simulink model "SimulacionControl9"  (R2022b)
settings: Solver=VariableStepAuto  StartTime=0.0  StopTime=20  RelTol=1e-3
undefined symbols (not defined in the file): Cdifuso9
libraries: fuzblock x1
settings Model: Creator=PC-LUISMIGUEL  LastModifiedBy=David

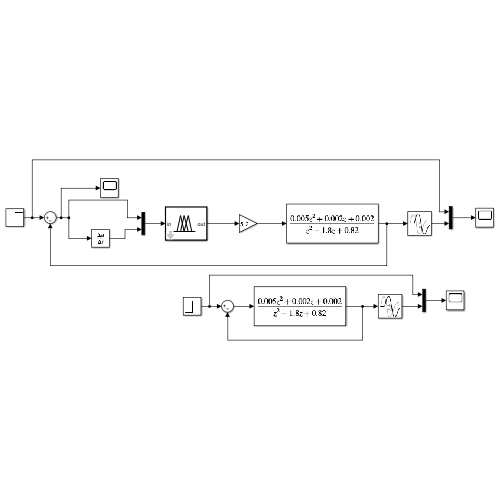
[thumbnail: Simulink's stored preview of the top-level diagram]
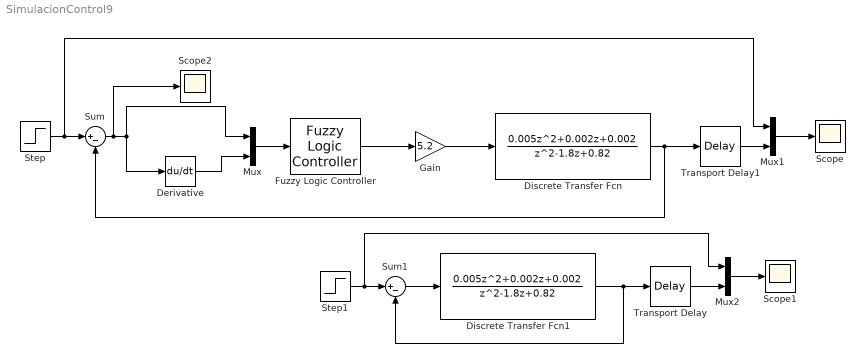
== system SimulacionControl9 ==
  Derivative : Derivative
  Discrete Transfer Fcn : DiscreteTransferFcn  Numerator=[0.005 0.002 0.002]  Denominator=[1 -1.8 0.82]  SampleTime=0.1
  Discrete Transfer Fcn1 : DiscreteTransferFcn  Numerator=[0.005 0.002 0.002]  Denominator=[1 -1.8 0.82]  SampleTime=0.1
  Fuzzy Logic Controller : fuzblock/Fuzzy Logic  Controller  FIS=[Cdifuso9]  OutputSampleNumber=101  DataType=double  FuzzifiedInputs=off  RuleFiringStrengths=off  RuleOutputs=off  AggregatedOutputs=off  SimulateUsing=Interpreted execution  OutOfRangeInputValueMessage=warning  NoRuleFiredMessage=warning  EmptyOutputFuzzySetMessage=warning
  Gain : Gain  Gain=5.2
  Mux : Mux  Inputs=2
  Mux1 : Mux  Inputs=2
  Mux2 : Mux  Inputs=2
  Scope : Scope
  Scope1 : Scope
  Scope2 : Scope
  Step : Step  SampleTime=0
  Step1 : Step  SampleTime=0
  Sum : Sum  Inputs=|+-
  Sum1 : Sum  Inputs=|+-
  Transport Delay : TransportDelay
  Transport Delay1 : TransportDelay
  wires:
  Step/1 -> Sum/1, Mux1/1
  Sum/1 -> Scope2/1, Mux/1, Derivative/1
  Derivative/1 -> Mux/2
  Mux/1 -> Fuzzy Logic Controller/1
  Discrete Transfer Fcn/1 -> Transport Delay1/1, Sum/2
  Mux1/1 -> Scope/1
  Discrete Transfer Fcn1/1 -> Sum1/2, Transport Delay/1
  Step1/1 -> Mux2/1, Sum1/1
  Sum1/1 -> Discrete Transfer Fcn1/1
  Transport Delay/1 -> Mux2/2
  Mux2/1 -> Scope1/1
  Transport Delay1/1 -> Mux1/2
  Fuzzy Logic Controller/1 -> Gain/1
  Gain/1 -> Discrete Transfer Fcn/1
